simulink model "dem_fs_inclass_activity_mar_6_2014"  (Simulink 7.9)
settings: Solver=ode5  SolverMode=SingleTasking  StartTime=0.0  StopTime=999999  FixedStep=0.000001  MaxStep=0.000001  RelTol=1e-3  AbsTol=1e-3
libraries: simulink x22
settings Model: Creator=kpayton  LastModifiedBy=okuu
settings DataIOCC: LimitDataPoints=off  SaveOutput=off  SaveTime=off
settings OptimizationCC: BlockReduction=off  BooleanDataType=off  InitFltsAndDblsToZero=on
settings DebuggingCC: SaveWithParameterizedLinksMsg=none  SignalResolutionControl=TryResolveAllWithWarning  SolverPrmCheckMsg=none  InheritedTsInSrcMsg=none  MultiTaskDSMMsg=warning  MultiTaskCondExecSysMsg=none  FcnCallInpInsideContextMsg=Use local settings  StrictBusMsg=None
settings HardwareCC: TargetUnknown=on
settings RTWCC: TemplateMakefile=grt_vc.tmf  IncludeERTFirstTime=on
settings GRTTargetCC: ModelReferenceCompliant=off  ParMdlRefBuildCompliant=off  CompOptLevelCompliant=off  ConcurrentExecutionCompliant=off  CombineOutputUpdateFcns=off  MatFileLogging=off  GRTInterface=on

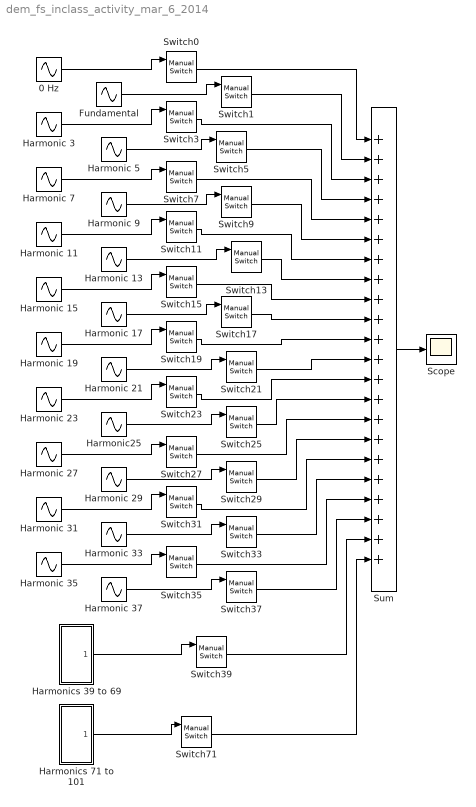
== system dem_fs_inclass_activity_mar_6_2014 ==
  " Switch0" : simulink/Signal Routing/Manual Switch  sw=1  action=0  varsize=off
  0 Hz : Sin  Amplitude=A  Frequency=w  Phase=P  mask(Sinusoidal source.){A=1/2}
      mask prompts: A "Amplitude:"
      mask help:
      | Sinusoidal source.
      | y = A sin(2*pi*f + phase)
      mask init:
      | w = 2 * pi * @2;P = @3 * (pi/180);
  Fundamental : Sin  Amplitude=A  Frequency=w  Phase=P  mask(Sinusoidal source.){A=(-4/pi^2)}
      mask prompts: A "Amplitude:"
      mask help:
      | Sinusoidal source.
      | y = A sin(2*pi*f + phase)
      mask init:
      | w = 2 * pi * @2;P = @3 * (pi/180);
  Harmonic 11 : Sin  Amplitude=A  Frequency=w  Phase=P  mask(Sinusoidal source.){A=(-2/(11*pi))}
      mask prompts: A "Amplitude:"
      mask help:
      | Sinusoidal source.
      | y = A sin(2*pi*f + phase)
      mask init:
      | w = 2 * pi * @2;P = @3 * (pi/180);
  Harmonic 13 : Sin  Amplitude=A  Frequency=w  Phase=P  mask(Sinusoidal source.){A=(2/(13*pi))}
      mask prompts: A "Amplitude:"
      mask help:
      | Sinusoidal source.
      | y = A sin(2*pi*f + phase)
      mask init:
      | w = 2 * pi * @2;P = @3 * (pi/180);
  Harmonic 15 : Sin  Amplitude=A  Frequency=w  Phase=P  mask(Sinusoidal source.){A=(-2/(15*pi))}
      mask prompts: A "Amplitude:"
      mask help:
      | Sinusoidal source.
      | y = A sin(2*pi*f + phase)
      mask init:
      | w = 2 * pi * @2;P = @3 * (pi/180);
  Harmonic 17 : Sin  Amplitude=A  Frequency=w  Phase=P  mask(Sinusoidal source.){A=(2/(17*pi))}
      mask prompts: A "Amplitude:"
      mask help:
      | Sinusoidal source.
      | y = A sin(2*pi*f + phase)
      mask init:
      | w = 2 * pi * @2;P = @3 * (pi/180);
  Harmonic 19 : Sin  Amplitude=A  Frequency=w  Phase=P  mask(Sinusoidal source.){A=(-2/(19*pi))}
      mask prompts: A "Amplitude:"
      mask help:
      | Sinusoidal source.
      | y = A sin(2*pi*f + phase)
      mask init:
      | w = 2 * pi * @2;P = @3 * (pi/180);
  Harmonic 21 : Sin  Amplitude=A  Frequency=w  Phase=P  mask(Sinusoidal source.){A=(2/(21*pi))}
      mask prompts: A "Amplitude:"
      mask help:
      | Sinusoidal source.
      | y = A sin(2*pi*f + phase)
      mask init:
      | w = 2 * pi * @2;P = @3 * (pi/180);
  Harmonic 23 : Sin  Amplitude=A  Frequency=w  Phase=P  mask(Sinusoidal source.){A=(-2/(23*pi))}
      mask prompts: A "Amplitude:"
      mask help:
      | Sinusoidal source.
      | y = A sin(2*pi*f + phase)
      mask init:
      | w = 2 * pi * @2;P = @3 * (pi/180);
  Harmonic 27 : Sin  Amplitude=A  Frequency=w  Phase=P  mask(Sinusoidal source.){A=(-2/(27*pi))}
      mask prompts: A "Amplitude:"
      mask help:
      | Sinusoidal source.
      | y = A sin(2*pi*f + phase)
      mask init:
      | w = 2 * pi * @2;P = @3 * (pi/180);
  Harmonic 29 : Sin  Amplitude=A  Frequency=w  Phase=P  mask(Sinusoidal source.){A=(2/(29*pi))}
      mask prompts: A "Amplitude:"
      mask help:
      | Sinusoidal source.
      | y = A sin(2*pi*f + phase)
      mask init:
      | w = 2 * pi * @2;P = @3 * (pi/180);
  Harmonic 3 : Sin  Amplitude=A  Frequency=w  Phase=P  mask(Sinusoidal source.){A=(-4/(9*pi^2))}
      mask prompts: A "Amplitude:"
      mask help:
      | Sinusoidal source.
      | y = A sin(2*pi*f + phase)
      mask init:
      | w = 2 * pi * @2;P = @3 * (pi/180);
  Harmonic 31 : Sin  Amplitude=A  Frequency=w  Phase=P  mask(Sinusoidal source.){A=(-2/(31*pi))}
      mask prompts: A "Amplitude:"
      mask help:
      | Sinusoidal source.
      | y = A sin(2*pi*f + phase)
      mask init:
      | w = 2 * pi * @2;P = @3 * (pi/180);
  Harmonic 33 : Sin  Amplitude=A  Frequency=w  Phase=P  mask(Sinusoidal source.){A=(2/(33*pi))}
      mask prompts: A "Amplitude:"
      mask help:
      | Sinusoidal source.
      | y = A sin(2*pi*f + phase)
      mask init:
      | w = 2 * pi * @2;P = @3 * (pi/180);
  Harmonic 35 : Sin  Amplitude=A  Frequency=w  Phase=P  mask(Sinusoidal source.){A=(-2/(35*pi))}
      mask prompts: A "Amplitude:"
      mask help:
      | Sinusoidal source.
      | y = A sin(2*pi*f + phase)
      mask init:
      | w = 2 * pi * @2;P = @3 * (pi/180);
  Harmonic 37 : Sin  Amplitude=A  Frequency=w  Phase=P  mask(Sinusoidal source.){A=(2/(37*pi))}
      mask prompts: A "Amplitude:"
      mask help:
      | Sinusoidal source.
      | y = A sin(2*pi*f + phase)
      mask init:
      | w = 2 * pi * @2;P = @3 * (pi/180);
  Harmonic 5 : Sin  Amplitude=A  Frequency=w  Phase=P  mask(Sinusoidal source.){A=(-4/(25*pi^2))}
      mask prompts: A "Amplitude:"
      mask help:
      | Sinusoidal source.
      | y = A sin(2*pi*f + phase)
      mask init:
      | w = 2 * pi * @2;P = @3 * (pi/180);
  Harmonic 7 : Sin  Amplitude=A  Frequency=w  Phase=P  mask(Sinusoidal source.){A=(-4/(49*pi^2))}
      mask prompts: A "Amplitude:"
      mask help:
      | Sinusoidal source.
      | y = A sin(2*pi*f + phase)
      mask init:
      | w = 2 * pi * @2;P = @3 * (pi/180);
  Harmonic 9 : Sin  Amplitude=A  Frequency=w  Phase=P  mask(Sinusoidal source.){A=(-4/(81*pi^2))}
      mask prompts: A "Amplitude:"
      mask help:
      | Sinusoidal source.
      | y = A sin(2*pi*f + phase)
      mask init:
      | w = 2 * pi * @2;P = @3 * (pi/180);
  Harmonic25 : Sin  Amplitude=A  Frequency=w  Phase=P  mask(Sinusoidal source.){A=(2/(25*pi))}
      mask prompts: A "Amplitude:"
      mask help:
      | Sinusoidal source.
      | y = A sin(2*pi*f + phase)
      mask init:
      | w = 2 * pi * @2;P = @3 * (pi/180);
  Harmonics 39 to 69 : Subsystem
  Harmonics 71 to 101 : Subsystem
  Scope : Scope
      settings: TickLabels=on  TimeRange=0.002000  YMin=-1.500000  YMax=1.500000
  Sum : Sum  Inputs=++++++++++++++++++++++  SaturateOnIntegerOverflow=on  InputSameDT=on  OutDataTypeStr=Inherit: Same as first input
  Switch{1,3,5,7,9} (5 alike) : simulink/Signal Routing/Manual Switch  sw=1  action=0  varsize=off
  Switch{11,13,15,17,19,21,23,25,27,29,31,33,35,37,39,71} (16 alike) : simulink/Signal Routing/Manual Switch  sw=0  action=0  varsize=off
  wires:
  Harmonic 23/1 -> Switch23/1
  Switch23/1 -> Sum/13
  Harmonic25/1 -> Switch25/1
  Harmonic 27/1 -> Switch27/1
  Switch27/1 -> Sum/15
  Harmonic 29/1 -> Switch29/1
  Harmonic 31/1 -> Switch31/1
  Switch31/1 -> Sum/17
  Harmonic 33/1 -> Switch33/1
  Harmonic 35/1 -> Switch35/1
  Harmonic 37/1 -> Switch37/1
  Harmonics 71 to 101/1(out_1) -> Switch71/1
  Switch71/1 -> Sum/22
  Harmonics 39 to 69/1(out_1) -> Switch39/1
  Harmonic 21/1 -> Switch21/1
  Harmonic 19/1 -> Switch19/1
  Switch19/1 -> Sum/11
  Harmonic 17/1 -> Switch17/1
  Switch17/1 -> Sum/10
  Harmonic 15/1 -> Switch15/1
  Harmonic 13/1 -> Switch13/1
  Switch11/1 -> Sum/7
  Harmonic 11/1 -> Switch11/1
  Harmonic 9/1 -> Switch9/1
  Switch9/1 -> Sum/6
  Switch7/1 -> Sum/5
  Harmonic 7/1 -> Switch7/1
  Switch5/1 -> Sum/4
  Harmonic 5/1 -> Switch5/1
  Harmonic 3/1 -> Switch3/1
  0 Hz/1 -> " Switch0"/1
  Switch3/1 -> Sum/3
  " Switch0"/1 -> Sum/1
  Switch1/1 -> Sum/2
  Fundamental/1 -> Switch1/1
  Switch39/1 -> Sum/21
  Switch37/1 -> Sum/20
  Switch35/1 -> Sum/19
  Switch33/1 -> Sum/18
  Switch29/1 -> Sum/16
  Switch25/1 -> Sum/14
  Switch21/1 -> Sum/12
  Sum/1 -> Scope/1
  Switch15/1 -> Sum/9
  Switch13/1 -> Sum/8

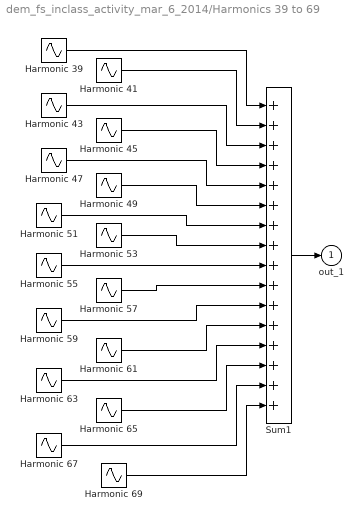
== system dem_fs_inclass_activity_mar_6_2014/Harmonics 39 to 69 ==
  Harmonic 39 : Sin  Amplitude=A  Frequency=w  Phase=P  mask(Sinusoidal source.){A=(-2/(39*pi))}
      mask prompts: A "Amplitude:"
      mask help:
      | Sinusoidal source.
      | y = A sin(2*pi*f + phase)
      mask init:
      | w = 2 * pi * @2;P = @3 * (pi/180);
  Harmonic 41 : Sin  Amplitude=A  Frequency=w  Phase=P  mask(Sinusoidal source.){A=(2/(41*pi))}
      mask prompts: A "Amplitude:"
      mask help:
      | Sinusoidal source.
      | y = A sin(2*pi*f + phase)
      mask init:
      | w = 2 * pi * @2;P = @3 * (pi/180);
  Harmonic 43 : Sin  Amplitude=A  Frequency=w  Phase=P  mask(Sinusoidal source.){A=(-2/(43*pi))}
      mask prompts: A "Amplitude:"
      mask help:
      | Sinusoidal source.
      | y = A sin(2*pi*f + phase)
      mask init:
      | w = 2 * pi * @2;P = @3 * (pi/180);
  Harmonic 45 : Sin  Amplitude=A  Frequency=w  Phase=P  mask(Sinusoidal source.){A=(2/(45*pi))}
      mask prompts: A "Amplitude:"
      mask help:
      | Sinusoidal source.
      | y = A sin(2*pi*f + phase)
      mask init:
      | w = 2 * pi * @2;P = @3 * (pi/180);
  Harmonic 47 : Sin  Amplitude=A  Frequency=w  Phase=P  mask(Sinusoidal source.){A=(-2/(47*pi))}
      mask prompts: A "Amplitude:"
      mask help:
      | Sinusoidal source.
      | y = A sin(2*pi*f + phase)
      mask init:
      | w = 2 * pi * @2;P = @3 * (pi/180);
  Harmonic 49 : Sin  Amplitude=A  Frequency=w  Phase=P  mask(Sinusoidal source.){A=(2/(49*pi))}
      mask prompts: A "Amplitude:"
      mask help:
      | Sinusoidal source.
      | y = A sin(2*pi*f + phase)
      mask init:
      | w = 2 * pi * @2;P = @3 * (pi/180);
  Harmonic 51 : Sin  Amplitude=A  Frequency=w  Phase=P  mask(Sinusoidal source.){A=(-2/(51*pi))}
      mask prompts: A "Amplitude:"
      mask help:
      | Sinusoidal source.
      | y = A sin(2*pi*f + phase)
      mask init:
      | w = 2 * pi * @2;P = @3 * (pi/180);
  Harmonic 53 : Sin  Amplitude=A  Frequency=w  Phase=P  mask(Sinusoidal source.){A=(2/(53*pi))}
      mask prompts: A "Amplitude:"
      mask help:
      | Sinusoidal source.
      | y = A sin(2*pi*f + phase)
      mask init:
      | w = 2 * pi * @2;P = @3 * (pi/180);
  Harmonic 55 : Sin  Amplitude=A  Frequency=w  Phase=P  mask(Sinusoidal source.){A=(-2/(55*pi))}
      mask prompts: A "Amplitude:"
      mask help:
      | Sinusoidal source.
      | y = A sin(2*pi*f + phase)
      mask init:
      | w = 2 * pi * @2;P = @3 * (pi/180);
  Harmonic 57 : Sin  Amplitude=A  Frequency=w  Phase=P  mask(Sinusoidal source.){A=(2/(57*pi))}
      mask prompts: A "Amplitude:"
      mask help:
      | Sinusoidal source.
      | y = A sin(2*pi*f + phase)
      mask init:
      | w = 2 * pi * @2;P = @3 * (pi/180);
  Harmonic 59 : Sin  Amplitude=A  Frequency=w  Phase=P  mask(Sinusoidal source.){A=(-2/(59*pi))}
      mask prompts: A "Amplitude:"
      mask help:
      | Sinusoidal source.
      | y = A sin(2*pi*f + phase)
      mask init:
      | w = 2 * pi * @2;P = @3 * (pi/180);
  Harmonic 61 : Sin  Amplitude=A  Frequency=w  Phase=P  mask(Sinusoidal source.){A=(2/(61*pi))}
      mask prompts: A "Amplitude:"
      mask help:
      | Sinusoidal source.
      | y = A sin(2*pi*f + phase)
      mask init:
      | w = 2 * pi * @2;P = @3 * (pi/180);
  Harmonic 63 : Sin  Amplitude=A  Frequency=w  Phase=P  mask(Sinusoidal source.){A=(-2/(63*pi))}
      mask prompts: A "Amplitude:"
      mask help:
      | Sinusoidal source.
      | y = A sin(2*pi*f + phase)
      mask init:
      | w = 2 * pi * @2;P = @3 * (pi/180);
  Harmonic 65 : Sin  Amplitude=A  Frequency=w  Phase=P  mask(Sinusoidal source.){A=(2/(65*pi))}
      mask prompts: A "Amplitude:"
      mask help:
      | Sinusoidal source.
      | y = A sin(2*pi*f + phase)
      mask init:
      | w = 2 * pi * @2;P = @3 * (pi/180);
  Harmonic 67 : Sin  Amplitude=A  Frequency=w  Phase=P  mask(Sinusoidal source.){A=(-2/(67*pi))}
      mask prompts: A "Amplitude:"
      mask help:
      | Sinusoidal source.
      | y = A sin(2*pi*f + phase)
      mask init:
      | w = 2 * pi * @2;P = @3 * (pi/180);
  Harmonic 69 : Sin  Amplitude=A  Frequency=w  Phase=P  mask(Sinusoidal source.){A=(2/(69*pi))}
      mask prompts: A "Amplitude:"
      mask help:
      | Sinusoidal source.
      | y = A sin(2*pi*f + phase)
      mask init:
      | w = 2 * pi * @2;P = @3 * (pi/180);
  Sum1 : Sum  Inputs=++++++++++++++++  SaturateOnIntegerOverflow=on  InputSameDT=on  OutDataTypeStr=Inherit: Same as first input
  out_1 : Outport  InitialOutput=0
  wires:
  Harmonic 69/1 -> Sum1/16
  Harmonic 67/1 -> Sum1/15
  Harmonic 65/1 -> Sum1/14
  Harmonic 63/1 -> Sum1/13
  Sum1/1 -> out_1/1
  Harmonic 39/1 -> Sum1/1
  Harmonic 41/1 -> Sum1/2
  Harmonic 43/1 -> Sum1/3
  Harmonic 45/1 -> Sum1/4
  Harmonic 47/1 -> Sum1/5
  Harmonic 49/1 -> Sum1/6
  Harmonic 51/1 -> Sum1/7
  Harmonic 53/1 -> Sum1/8
  Harmonic 55/1 -> Sum1/9
  Harmonic 57/1 -> Sum1/10
  Harmonic 59/1 -> Sum1/11
  Harmonic 61/1 -> Sum1/12

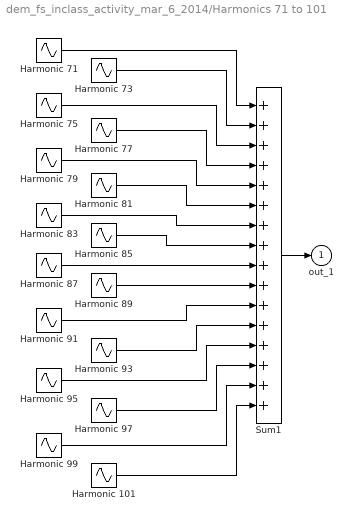
== system dem_fs_inclass_activity_mar_6_2014/Harmonics 71 to 101 ==
  Harmonic 101 : Sin  Amplitude=A  Frequency=w  Phase=P  mask(Sinusoidal source.){A=(2/(101*pi))}
      mask prompts: A "Amplitude:"
      mask help:
      | Sinusoidal source.
      | y = A sin(2*pi*f + phase)
      mask init:
      | w = 2 * pi * @2;P = @3 * (pi/180);
  Harmonic 71 : Sin  Amplitude=A  Frequency=w  Phase=P  mask(Sinusoidal source.){A=(-2/(71*pi))}
      mask prompts: A "Amplitude:"
      mask help:
      | Sinusoidal source.
      | y = A sin(2*pi*f + phase)
      mask init:
      | w = 2 * pi * @2;P = @3 * (pi/180);
  Harmonic 73 : Sin  Amplitude=A  Frequency=w  Phase=P  mask(Sinusoidal source.){A=(2/(73*pi))}
      mask prompts: A "Amplitude:"
      mask help:
      | Sinusoidal source.
      | y = A sin(2*pi*f + phase)
      mask init:
      | w = 2 * pi * @2;P = @3 * (pi/180);
  Harmonic 75 : Sin  Amplitude=A  Frequency=w  Phase=P  mask(Sinusoidal source.){A=(-2/(75*pi))}
      mask prompts: A "Amplitude:"
      mask help:
      | Sinusoidal source.
      | y = A sin(2*pi*f + phase)
      mask init:
      | w = 2 * pi * @2;P = @3 * (pi/180);
  Harmonic 77 : Sin  Amplitude=A  Frequency=w  Phase=P  mask(Sinusoidal source.){A=(2/(77*pi))}
      mask prompts: A "Amplitude:"
      mask help:
      | Sinusoidal source.
      | y = A sin(2*pi*f + phase)
      mask init:
      | w = 2 * pi * @2;P = @3 * (pi/180);
  Harmonic 79 : Sin  Amplitude=A  Frequency=w  Phase=P  mask(Sinusoidal source.){A=(-2/(79*pi))}
      mask prompts: A "Amplitude:"
      mask help:
      | Sinusoidal source.
      | y = A sin(2*pi*f + phase)
      mask init:
      | w = 2 * pi * @2;P = @3 * (pi/180);
  Harmonic 81 : Sin  Amplitude=A  Frequency=w  Phase=P  mask(Sinusoidal source.){A=(2/(81*pi))}
      mask prompts: A "Amplitude:"
      mask help:
      | Sinusoidal source.
      | y = A sin(2*pi*f + phase)
      mask init:
      | w = 2 * pi * @2;P = @3 * (pi/180);
  Harmonic 83 : Sin  Amplitude=A  Frequency=w  Phase=P  mask(Sinusoidal source.){A=(-2/(83*pi))}
      mask prompts: A "Amplitude:"
      mask help:
      | Sinusoidal source.
      | y = A sin(2*pi*f + phase)
      mask init:
      | w = 2 * pi * @2;P = @3 * (pi/180);
  Harmonic 85 : Sin  Amplitude=A  Frequency=w  Phase=P  mask(Sinusoidal source.){A=(2/(85*pi))}
      mask prompts: A "Amplitude:"
      mask help:
      | Sinusoidal source.
      | y = A sin(2*pi*f + phase)
      mask init:
      | w = 2 * pi * @2;P = @3 * (pi/180);
  Harmonic 87 : Sin  Amplitude=A  Frequency=w  Phase=P  mask(Sinusoidal source.){A=(-2/(87*pi))}
      mask prompts: A "Amplitude:"
      mask help:
      | Sinusoidal source.
      | y = A sin(2*pi*f + phase)
      mask init:
      | w = 2 * pi * @2;P = @3 * (pi/180);
  Harmonic 89 : Sin  Amplitude=A  Frequency=w  Phase=P  mask(Sinusoidal source.){A=(2/(89*pi))}
      mask prompts: A "Amplitude:"
      mask help:
      | Sinusoidal source.
      | y = A sin(2*pi*f + phase)
      mask init:
      | w = 2 * pi * @2;P = @3 * (pi/180);
  Harmonic 91 : Sin  Amplitude=A  Frequency=w  Phase=P  mask(Sinusoidal source.){A=(-2/(91*pi))}
      mask prompts: A "Amplitude:"
      mask help:
      | Sinusoidal source.
      | y = A sin(2*pi*f + phase)
      mask init:
      | w = 2 * pi * @2;P = @3 * (pi/180);
  Harmonic 93 : Sin  Amplitude=A  Frequency=w  Phase=P  mask(Sinusoidal source.){A=(2/(93*pi))}
      mask prompts: A "Amplitude:"
      mask help:
      | Sinusoidal source.
      | y = A sin(2*pi*f + phase)
      mask init:
      | w = 2 * pi * @2;P = @3 * (pi/180);
  Harmonic 95 : Sin  Amplitude=A  Frequency=w  Phase=P  mask(Sinusoidal source.){A=(-2/(95*pi))}
      mask prompts: A "Amplitude:"
      mask help:
      | Sinusoidal source.
      | y = A sin(2*pi*f + phase)
      mask init:
      | w = 2 * pi * @2;P = @3 * (pi/180);
  Harmonic 97 : Sin  Amplitude=A  Frequency=w  Phase=P  mask(Sinusoidal source.){A=(2/(97*pi))}
      mask prompts: A "Amplitude:"
      mask help:
      | Sinusoidal source.
      | y = A sin(2*pi*f + phase)
      mask init:
      | w = 2 * pi * @2;P = @3 * (pi/180);
  Harmonic 99 : Sin  Amplitude=A  Frequency=w  Phase=P  mask(Sinusoidal source.){A=(-2/(99*pi))}
      mask prompts: A "Amplitude:"
      mask help:
      | Sinusoidal source.
      | y = A sin(2*pi*f + phase)
      mask init:
      | w = 2 * pi * @2;P = @3 * (pi/180);
  Sum1 : Sum  Inputs=++++++++++++++++  SaturateOnIntegerOverflow=on  InputSameDT=on  OutDataTypeStr=Inherit: Same as first input
  out_1 : Outport  InitialOutput=0
  wires:
  Harmonic 101/1 -> Sum1/16
  Harmonic 99/1 -> Sum1/15
  Harmonic 97/1 -> Sum1/14
  Harmonic 95/1 -> Sum1/13
  Sum1/1 -> out_1/1
  Harmonic 71/1 -> Sum1/1
  Harmonic 73/1 -> Sum1/2
  Harmonic 75/1 -> Sum1/3
  Harmonic 77/1 -> Sum1/4
  Harmonic 79/1 -> Sum1/5
  Harmonic 81/1 -> Sum1/6
  Harmonic 83/1 -> Sum1/7
  Harmonic 85/1 -> Sum1/8
  Harmonic 87/1 -> Sum1/9
  Harmonic 89/1 -> Sum1/10
  Harmonic 91/1 -> Sum1/11
  Harmonic 93/1 -> Sum1/12
